simulink model "Practica1seminario"  (R2017b)
settings: Solver=ode23  StartTime=0.0  StopTime=200  RelTol=1e-3
settings Model: Creator=Charles  LastModifiedBy=Charles

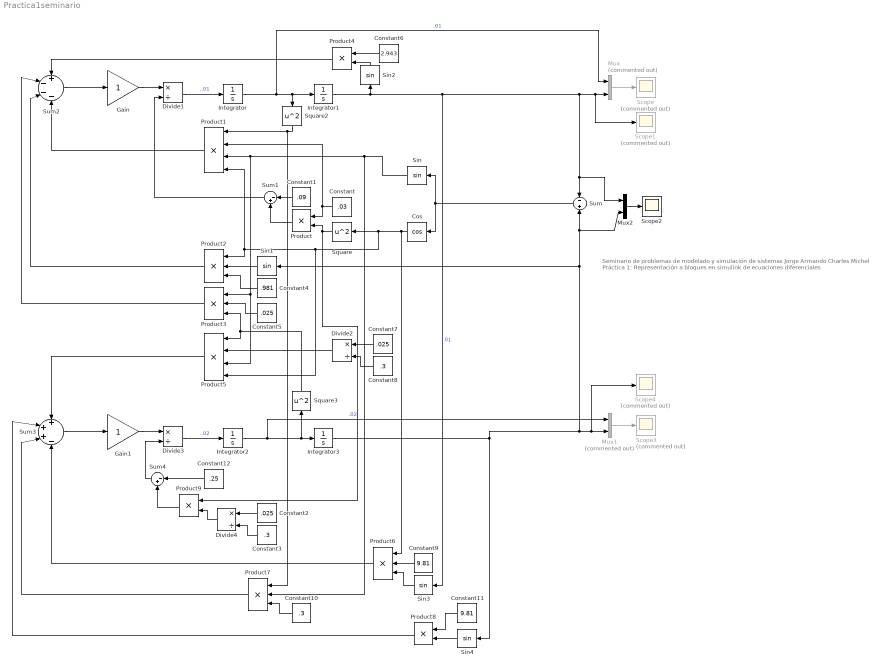
== system Practica1seminario ==
  note: Seminario de problemas de modelado y simulación de sistemas
      |
      | Jorge Armando Charles Michel
      |
      | Práctica 1: Representación a bloques en simulink de ecuaciones diferenciales
  Constant : Constant  Value=.03
  Constant1 : Constant  Value=.09
  Constant10 : Constant  Value=.3
  Constant11 : Constant  Value=9.81
  Constant12 : Constant  Value=.25
  Constant2 : Constant  Value=.025
  Constant3 : Constant  Value=.3
  Constant4 : Constant  Value=.981
  Constant5 : Constant  Value=.025
  Constant6 : Constant  Value=2.943
  Constant7 : Constant  Value=.025
  Constant8 : Constant  Value=.3
  Constant9 : Constant  Value=9.81
  Cos : Trigonometry  Operator=cos
  Divide{1..4} (4 alike) : Product  Inputs=*/
  Gain : Gain
  Gain1 : Gain
  Integrator : Integrator
  Integrator1 : Integrator
  Integrator2 : Integrator
  Integrator3 : Integrator  InitialCondition=0.610865
  Mux : Mux  Commented=on  Inputs=2
  Mux1 : Mux  Commented=on  Inputs=2
  Mux2 : Mux  Inputs=2
  Product{,4,8..9} (4 alike) : Product
  Product1 : Product  Inputs=4
  Product{2..3,6..7} (4 alike) : Product  Inputs=3
  Product5 : Product  Inputs=4
  Scope{,1,3..4} (4 alike) : Scope  Commented=on
  Scope2 : Scope
  Sin{,1..4} (5 alike) : Trigonometry
  Square : Math  Operator=square  RndMeth=Zero  SaturateOnIntegerOverflow=on
  Square2 : Math  Operator=square  RndMeth=Zero  SaturateOnIntegerOverflow=on
  Square3 : Math  Operator=square  RndMeth=Zero  SaturateOnIntegerOverflow=on
  Sum : Sum  Inputs=-+
  Sum1 : Sum  Inputs=|-+
  Sum2 : Sum  Inputs=+---
  Sum3 : Sum  Inputs=+++-
  Sum4 : Sum  Inputs=|-+
  wires:
  Gain/1 -> Divide1/1
  Integrator/1 -> Mux/1, Square2/1, Integrator1/1  ".01"
  Integrator1/1 -> Sin2/1, Sin3/1, Scope1/1, Mux/2, Mux2/1, Sum/1  "01"
  Integrator2/1 -> Mux1/1, Square3/1, Integrator3/1  ".02"
  Integrator3/1 -> Scope4/1, Mux1/2, Sin1/1, Mux2/2, Sum/2, Sin4/1
  Gain1/1 -> Divide3/1
  Sum/1 -> Sin/1, Cos/1
  Cos/1 -> Product5/4, Product2/1, Product1/4, Square/1, Product6/1
  Sin/1 -> Product5/3, Product3/1, Product1/3, Product7/2
  Square/1 -> Product9/1, Product/2
  Constant/1 -> Product/1, Product1/2
  Constant1/1 -> Sum1/1
  Product/1 -> Sum1/2
  Sum1/1 -> Divide1/2
  Divide1/1 -> Integrator/1  "..01"
  Sum2/1 -> Gain/1
  Square2/1 -> Product1/1, Product7/1
  Product1/1 -> Sum2/4
  Sin1/1 -> Product2/2
  Constant4/1 -> Product2/3
  Product2/1 -> Sum2/3
  Constant5/1 -> Product3/2
  Square3/1 -> Product5/1, Product3/3
  Product3/1 -> Sum2/2
  Sin2/1 -> Product4/2
  Constant6/1 -> Product4/1
  Product4/1 -> Sum2/1
  Sum3/1 -> Gain1/1
  Constant8/1 -> Divide2/2
  Constant7/1 -> Divide2/1
  Divide2/1 -> Product5/2
  Product5/1 -> Sum3/1
  Sin3/1 -> Product6/3
  Constant9/1 -> Product6/2
  Constant10/1 -> Product7/3
  Product7/1 -> Sum3/3
  Product6/1 -> Sum3/4
  Sin4/1 -> Product8/2
  Constant11/1 -> Product8/1
  Product8/1 -> Sum3/2
  Mux/1 -> Scope/1
  Mux1/1 -> Scope3/1
  Divide3/1 -> Integrator2/1  "..02"
  Constant2/1 -> Divide4/1
  Constant3/1 -> Divide4/2
  Divide4/1 -> Product9/2
  Product9/1 -> Sum4/2
  Constant12/1 -> Sum4/1
  Sum4/1 -> Divide3/2
  Mux2/1 -> Scope2/1
